simulink model "MMC_THRTN"  (R2023b)
settings: Solver=VariableStepAuto  StartTime=0.0  StopTime=0.1  RelTol=1e-3
undefined symbols (not defined in the file): k
libraries: spsMosfetLib x48, spsSeriesRLCBranchLib x25, spsDCVoltageSourceLib x2, spsGroundLib x2, spsVoltageMeasurementLib x1, sps_lib x1
settings Model: Creator=ganeshguguloth  LastModifiedBy=ganeshguguloth

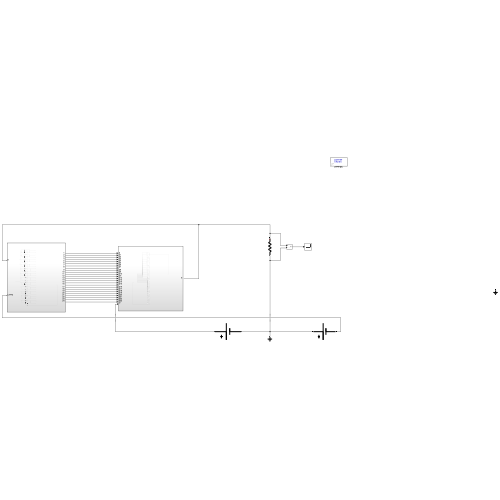
[thumbnail: Simulink's stored preview of the top-level diagram]
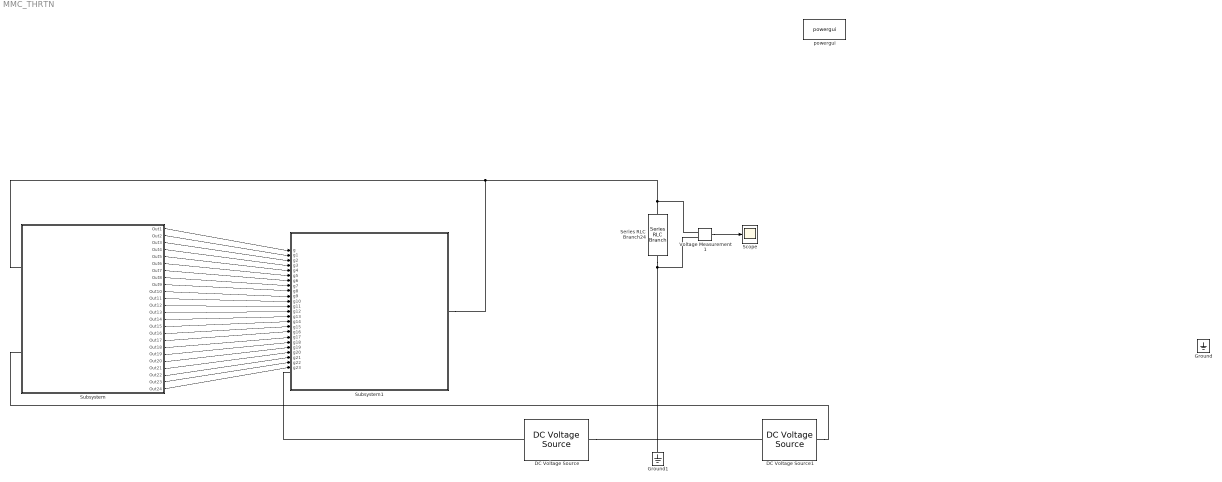
== system MMC_THRTN ==
  DC Voltage Source : spsDCVoltageSourceLib/DC Voltage Source  Amplitude=100  Measurements=None
  DC Voltage Source1 : spsDCVoltageSourceLib/DC Voltage Source  Amplitude=100  Measurements=None
  Ground : spsGroundLib/Ground  LConnTagsString=a
  Ground1 : spsGroundLib/Ground  LConnTagsString=a
  Scope : Scope
  Series RLC Branch24 : spsSeriesRLCBranchLib/Series RLC Branch  LConnTagsString=__new0  RConnTagsString=__new0  BranchType=R  Resistance=15000  Inductance=1e-3  SetiL0=off  InitialCurrent=0  Capacitance=1e-6  Setx0=off  InitialVoltage=0  Measurements=None
  Subsystem : Subsystem
  Subsystem1 : Subsystem
  Voltage Measurement1 : spsVoltageMeasurementLib/Voltage Measurement  PhasorSimulation=off  OutputType=Complex  PSBequivalent=0
  powergui : sps_lib/powergui  Priority=1  SimulationMode=Discrete  SampleTime=50e-6  frequency=60  Iterations=50  frequencyindice=0  Pbase=100e6  ErrMax=1e-4  UnitsV=kV  UnitsW=MW  buscounter=0  FunctionMessages=off  echomessages=off  EnableUseOfTLC=off  CurrentSourceSwitches=off  DisableSnubberDevices=off  DisableRonSwitches=off  DisableVfSwitches=off  DisplayEquations=off  AutomaticDiscreteSolvers=off  SolverType=Tustin/Backward Euler (TBE)  Interpol=off  ExternalGateDelay=off  methode=off  Ts=100  x0status=blocks  SPID=on  SwTol=0  HookPort=off  NonlinearTolerance=1e-4  nMaxIteration=100  ContinueOnMaxIteration=off  RestoreLinks=warning  ResistiveCurrentMeasurement=off  Frange=[0:2:500]  Ylog=off  Xlog=on  ShowGrid=off  save=off  variable=ZData  structure=0  ZoomFFT=off  StartTime=0.0  cycles=1  DisplayStyle=1  fundamental=60  FreqAxis=off  MaxFrequency=1000  frequencyindicesteady=1  RmsSteady=1  display=off
  wires:
  Voltage Measurement1/1 -> Scope/1
  Subsystem/1(Out1) -> Subsystem1/1(g)
  Subsystem/2(Out2) -> Subsystem1/2(g1)
  Subsystem/3(Out3) -> Subsystem1/3(g2)
  Subsystem/4(Out4) -> Subsystem1/4(g3)
  Subsystem/5(Out5) -> Subsystem1/5(g4)
  Subsystem/6(Out6) -> Subsystem1/6(g5)
  Subsystem/7(Out7) -> Subsystem1/7(g6)
  Subsystem/8(Out8) -> Subsystem1/8(g7)
  Subsystem/9(Out9) -> Subsystem1/9(g8)
  Subsystem/10(Out10) -> Subsystem1/10(g9)
  Subsystem/11(Out11) -> Subsystem1/11(g10)
  Subsystem/12(Out12) -> Subsystem1/12(g11)
  Subsystem/13(Out13) -> Subsystem1/13(g12)
  Subsystem/14(Out14) -> Subsystem1/14(g13)
  Subsystem/15(Out15) -> Subsystem1/15(g14)
  Subsystem/16(Out16) -> Subsystem1/16(g15)
  Subsystem/17(Out17) -> Subsystem1/17(g16)
  Subsystem/18(Out18) -> Subsystem1/18(g17)
  Subsystem/19(Out19) -> Subsystem1/19(g18)
  Subsystem/20(Out20) -> Subsystem1/20(g19)
  Subsystem/21(Out21) -> Subsystem1/21(g20)
  Subsystem/22(Out22) -> Subsystem1/22(g21)
  Subsystem/23(Out23) -> Subsystem1/23(g22)
  Subsystem/24(Out24) -> Subsystem1/24(g23)
  connections:
  DC Voltage Source1/LConn1 -- Subsystem/LConn2
  Voltage Measurement1/LConn1 -- Series RLC Branch24/LConn1 -- Subsystem1/RConn1 -- Subsystem/LConn1
  DC Voltage Source/RConn1 -- Subsystem1/LConn1
  Voltage Measurement1/LConn2 -- Series RLC Branch24/RConn1 -- DC Voltage Source1/RConn1 -- Ground1/LConn1 -- DC Voltage Source/LConn1

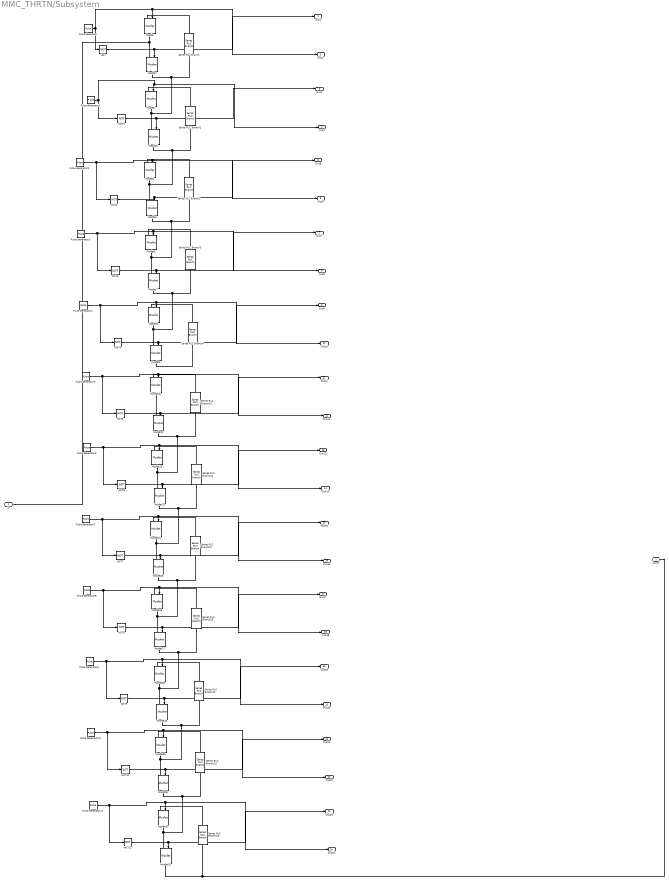
== system MMC_THRTN/Subsystem ==
  Mosfet{,1..9,20..33} (24 alike) : spsMosfetLib/Mosfet  Ron=0.1  Lon=0  Rd=0.01  Vfd=0  IC=0  Rs=1e5  Cs=inf  Measurements=off
  NOT{,1..11} (12 alike) : Logic  Operator=NOT  AllPortsSameDT=off  OutDataTypeStr=boolean
  Pulse Generator : DiscretePulseGenerator  PulseType=Time based  Period=0.02  PulseWidth=50  PhaseDelay=6e-3
  Pulse Generator1 : DiscretePulseGenerator  PulseType=Time based  Period=0.02  PulseWidth=50  PhaseDelay=5e-3
  Pulse Generator10 : DiscretePulseGenerator  PulseType=Time based  Period=0.02  PulseWidth=50  PhaseDelay=8e-3
  Pulse Generator11 : DiscretePulseGenerator  PulseType=Time based  Period=0.02  PulseWidth=50  PhaseDelay=7e-3
  Pulse Generator2 : DiscretePulseGenerator  PulseType=Time based  Period=0.02  PulseWidth=50  PhaseDelay=4e-3
  Pulse Generator3 : DiscretePulseGenerator  PulseType=Time based  Period=0.02  PulseWidth=50  PhaseDelay=3e-3
  Pulse Generator4 : DiscretePulseGenerator  PulseType=Time based  Period=0.02  PulseWidth=50  PhaseDelay=2e-3
  Pulse Generator5 : DiscretePulseGenerator  PulseType=Time based  Period=0.02  PulseWidth=50  PhaseDelay=1e-3
  Pulse Generator6 : DiscretePulseGenerator  PulseType=Time based  Period=0.02  PulseWidth=50  PhaseDelay=12e-3
  Pulse Generator7 : DiscretePulseGenerator  PulseType=Time based  Period=0.02  PulseWidth=50  PhaseDelay=11e-3
  Pulse Generator8 : DiscretePulseGenerator  PulseType=Time based  Period=0.02  PulseWidth=50  PhaseDelay=10e-3
  Pulse Generator9 : DiscretePulseGenerator  PulseType=Time based  Period=0.02  PulseWidth=50  PhaseDelay=9e-3
  Series RLC Branch{,1..4,10..16} (12 alike) : spsSeriesRLCBranchLib/Series RLC Branch  LConnTagsString=__new0  RConnTagsString=__new0  BranchType=C  Resistance=1  Inductance=1e-3  SetiL0=off  InitialCurrent=0  Capacitance=k  Setx0=off  InitialVoltage=0  Measurements=None
  D : PMIOPort  Side=Left
  Conn2 : PMIOPort  Port=2  Side=Left
  Out1 : Outport
  Out2 : Outport  Port=2
  Out3 : Outport  Port=3
  Out4 : Outport  Port=4
  Out5 : Outport  Port=5
  Out6 : Outport  Port=6
  Out7 : Outport  Port=7
  Out8 : Outport  Port=8
  Out9 : Outport  Port=9
  Out10 : Outport  Port=10
  Out11 : Outport  Port=11
  Out12 : Outport  Port=12
  Out13 : Outport  Port=13
  Out14 : Outport  Port=14
  Out15 : Outport  Port=15
  Out16 : Outport  Port=16
  Out17 : Outport  Port=17
  Out18 : Outport  Port=18
  Out19 : Outport  Port=19
  Out20 : Outport  Port=20
  Out21 : Outport  Port=21
  Out22 : Outport  Port=22
  Out23 : Outport  Port=23
  Out24 : Outport  Port=24
  wires:
  Pulse Generator8/1 -> NOT8/1, Out18/1, Mosfet26/1
  NOT6/1 -> Out13/1, Mosfet23/1
  NOT3/1 -> Out7/1, Mosfet7/1
  Pulse Generator5/1 -> Out12/1, Mosfet20/1, NOT5/1
  Pulse Generator4/1 -> NOT4/1, Out10/1, Mosfet8/1
  NOT10/1 -> Out21/1, Mosfet31/1
  NOT8/1 -> Out17/1, Mosfet27/1
  Pulse Generator2/1 -> NOT2/1, Out6/1, Mosfet4/1
  NOT7/1 -> Out15/1, Mosfet25/1
  NOT11/1 -> Out23/1, Mosfet33/1
  NOT/1 -> Out1/1, Mosfet1/1
  Pulse Generator3/1 -> Out8/1, Mosfet6/1, NOT3/1
  Pulse Generator1/1 -> Out4/1, Mosfet2/1, NOT1/1
  NOT4/1 -> Out9/1, Mosfet9/1
  NOT9/1 -> Out19/1, Mosfet29/1
  NOT1/1 -> Out3/1, Mosfet3/1
  Pulse Generator11/1 -> Out24/1, Mosfet32/1, NOT11/1
  NOT2/1 -> Out5/1, Mosfet5/1
  Pulse Generator6/1 -> NOT6/1, Out14/1, Mosfet22/1
  Pulse Generator/1 -> Out2/1, Mosfet/1, NOT/1
  Pulse Generator10/1 -> NOT10/1, Out22/1, Mosfet30/1
  NOT5/1 -> Out11/1, Mosfet21/1
  Pulse Generator7/1 -> Out16/1, Mosfet24/1, NOT7/1
  Pulse Generator9/1 -> Out20/1, Mosfet28/1, NOT9/1
  connections:
  Series RLC Branch14/LConn1 -- Mosfet28/LConn1
  Series RLC Branch13/LConn1 -- Mosfet26/LConn1
  Series RLC Branch12/LConn1 -- Mosfet24/LConn1
  Mosfet20/RConn1 -- Mosfet21/LConn1
  Mosfet21/RConn1 -- Mosfet23/LConn1 -- Mosfet22/RConn1 -- Series RLC Branch10/RConn1
  Series RLC Branch10/LConn1 -- Mosfet20/LConn1
  Series RLC Branch4/LConn1 -- Mosfet8/LConn1
  Mosfet27/LConn1 -- Mosfet25/RConn1 -- Series RLC Branch12/RConn1 -- Mosfet26/RConn1
  Mosfet30/RConn1 -- Series RLC Branch14/RConn1 -- Mosfet29/RConn1 -- Mosfet31/LConn1
  Series RLC Branch3/LConn1 -- Mosfet6/LConn1
  Series RLC Branch2/RConn1 -- Mosfet5/RConn1 -- Mosfet6/RConn1 -- Mosfet7/LConn1
  Series RLC Branch1/LConn1 -- Mosfet2/LConn1
  Series RLC Branch16/LConn1 -- Mosfet32/LConn1
  Mosfet9/RConn1 -- Series RLC Branch4/RConn1
  Mosfet23/RConn1 -- Mosfet25/LConn1 -- Mosfet24/RConn1 -- Series RLC Branch11/RConn1
  Mosfet33/LConn1 -- Mosfet31/RConn1 -- Series RLC Branch15/RConn1 -- Mosfet32/RConn1
  Mosfet2/RConn1 -- Series RLC Branch/RConn1 -- Mosfet1/RConn1 -- Mosfet3/LConn1
  Series RLC Branch/LConn1 -- Mosfet/LConn1
  Mosfet8/RConn1 -- Series RLC Branch3/RConn1 -- Mosfet7/RConn1 -- Mosfet9/LConn1
  Mosfet33/RConn1 -- Conn2/RConn1 -- Series RLC Branch16/RConn1
  Mosfet27/RConn1 -- Mosfet29/LConn1 -- Mosfet28/RConn1 -- Series RLC Branch13/RConn1
  Mosfet4/RConn1 -- Series RLC Branch1/RConn1 -- Mosfet3/RConn1 -- Mosfet5/LConn1
  Series RLC Branch2/LConn1 -- Mosfet4/LConn1
  Series RLC Branch11/LConn1 -- Mosfet22/LConn1
  Series RLC Branch15/LConn1 -- Mosfet30/LConn1
  Mosfet/RConn1 -- D/RConn1 -- Mosfet1/LConn1

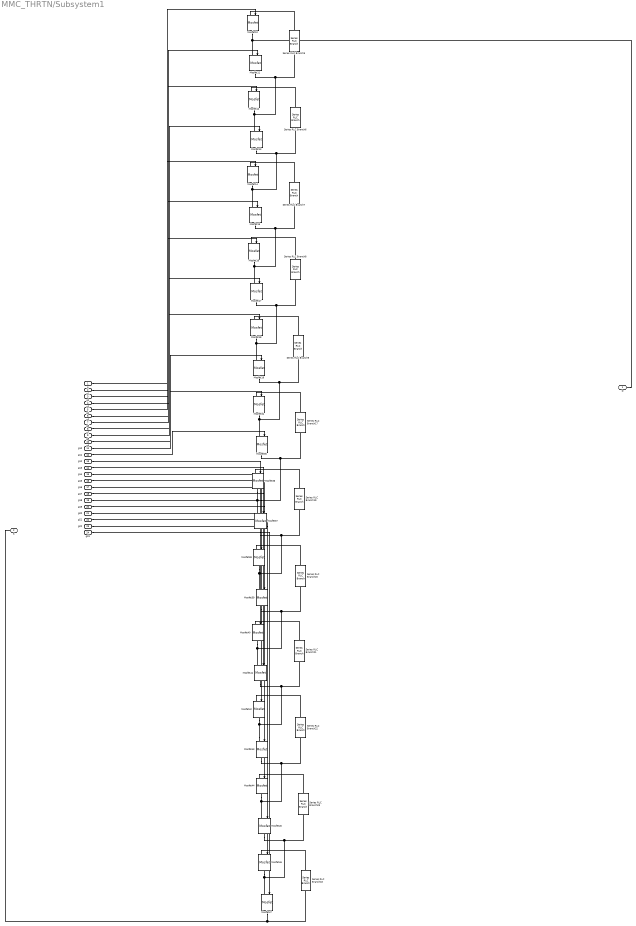
== system MMC_THRTN/Subsystem1 ==
  g : Inport
  g1 : Inport  Port=2
  g2 : Inport  Port=3
  g3 : Inport  Port=4
  g4 : Inport  Port=5
  g5 : Inport  Port=6
  g6 : Inport  Port=7
  g7 : Inport  Port=8
  g8 : Inport  Port=9
  g9 : Inport  Port=10
  g10 : Inport  Port=11
  g11 : Inport  Port=12
  g12 : Inport  Port=13
  g13 : Inport  Port=14
  g14 : Inport  Port=15
  g15 : Inport  Port=16
  g16 : Inport  Port=17
  g17 : Inport  Port=18
  g18 : Inport  Port=19
  g19 : Inport  Port=20
  g20 : Inport  Port=21
  g21 : Inport  Port=22
  g22 : Inport  Port=23
  g23 : Inport  Port=24
  Mosfet{10..19,34..47} (24 alike) : spsMosfetLib/Mosfet  Ron=0.1  Lon=0  Rd=0.01  Vfd=0  IC=0  Rs=1e5  Cs=inf  Measurements=off
  Series RLC Branch{5..9,17..23} (12 alike) : spsSeriesRLCBranchLib/Series RLC Branch  LConnTagsString=__new0  RConnTagsString=__new0  BranchType=C  Resistance=1  Inductance=1e-3  SetiL0=off  InitialCurrent=0  Capacitance=k  Setx0=off  InitialVoltage=0  Measurements=None
  D : PMIOPort  Side=Left
  S : PMIOPort  Port=2  Side=Right
  wires:
  g23/1 -> Mosfet47/1
  g22/1 -> Mosfet46/1
  g13/1 -> Mosfet37/1
  g5/1 -> Mosfet15/1
  g4/1 -> Mosfet14/1
  g3/1 -> Mosfet13/1
  g2/1 -> Mosfet12/1
  g18/1 -> Mosfet42/1
  g16/1 -> Mosfet40/1
  g8/1 -> Mosfet18/1
  g14/1 -> Mosfet38/1
  g7/1 -> Mosfet17/1
  g1/1 -> Mosfet11/1
  g12/1 -> Mosfet36/1
  g11/1 -> Mosfet35/1
  g21/1 -> Mosfet45/1
  g/1 -> Mosfet10/1
  g10/1 -> Mosfet34/1
  g17/1 -> Mosfet41/1
  g9/1 -> Mosfet19/1
  g20/1 -> Mosfet44/1
  g15/1 -> Mosfet39/1
  g6/1 -> Mosfet16/1
  g19/1 -> Mosfet43/1
  connections:
  Mosfet36/RConn1 -- Series RLC Branch17/RConn1 -- Mosfet35/RConn1 -- Mosfet37/LConn1
  Series RLC Branch23/RConn1 -- Mosfet45/RConn1 -- Mosfet46/RConn1 -- Mosfet47/LConn1
  Series RLC Branch8/LConn1 -- Mosfet16/LConn1
  Series RLC Branch6/LConn1 -- Mosfet12/LConn1
  Series RLC Branch17/LConn1 -- Mosfet34/LConn1
  Series RLC Branch5/LConn1 -- Mosfet10/LConn1
  Mosfet43/RConn1 -- Mosfet45/LConn1 -- Mosfet44/RConn1 -- Series RLC Branch22/RConn1
  Mosfet39/RConn1 -- Mosfet41/LConn1 -- Mosfet40/RConn1 -- Series RLC Branch20/RConn1
  Series RLC Branch7/LConn1 -- Mosfet14/LConn1
  Series RLC Branch22/LConn1 -- Mosfet42/LConn1
  Series RLC Branch19/LConn1 -- Mosfet36/LConn1
  Series RLC Branch9/LConn1 -- Mosfet18/LConn1
  Series RLC Branch20/LConn1 -- Mosfet38/LConn1
  Mosfet15/RConn1 -- Mosfet17/LConn1 -- Mosfet16/RConn1 -- Series RLC Branch7/RConn1
  Series RLC Branch8/RConn1 -- Mosfet17/RConn1 -- Mosfet18/RConn1 -- Mosfet19/LConn1
  Mosfet37/RConn1 -- Mosfet39/LConn1 -- Mosfet38/RConn1 -- Series RLC Branch19/RConn1
  Mosfet34/RConn1 -- Series RLC Branch9/RConn1 -- Mosfet19/RConn1 -- Mosfet35/LConn1
  Series RLC Branch21/LConn1 -- Mosfet40/LConn1
  Series RLC Branch5/RConn1 -- Mosfet11/RConn1 -- Mosfet12/RConn1 -- Mosfet13/LConn1
  Mosfet10/RConn1 -- D/RConn1 -- Mosfet11/LConn1
  Series RLC Branch23/LConn1 -- Mosfet44/LConn1
  Series RLC Branch6/RConn1 -- Mosfet13/RConn1 -- Mosfet14/RConn1 -- Mosfet15/LConn1
  Series RLC Branch18/LConn1 -- Mosfet46/LConn1
  Mosfet47/RConn1 -- Series RLC Branch18/RConn1 -- S/RConn1
  Mosfet43/LConn1 -- Mosfet41/RConn1 -- Series RLC Branch21/RConn1 -- Mosfet42/RConn1
